simulink model "specifications"  (R2019b)
settings: Solver=FixedStepAuto  StartTime=0.0  StopTime=10.0  FixedStep=fixedStepSize  RelTol=1e-3
settings Model: Creator=JEDDELAN  LastModifiedBy=JEDDELAN
settings DataIOCC: ReturnWorkspaceOutputs=off
settings DebuggingCC: ArithmeticOperatorsInVariantConditions=warning
settings SFSimCC: SimUseLocalCustomCode=off  CustomCodeUndefinedFunction=UseInterfaceOnly
settings RTWCC: RTWUseLocalCustomCode=off

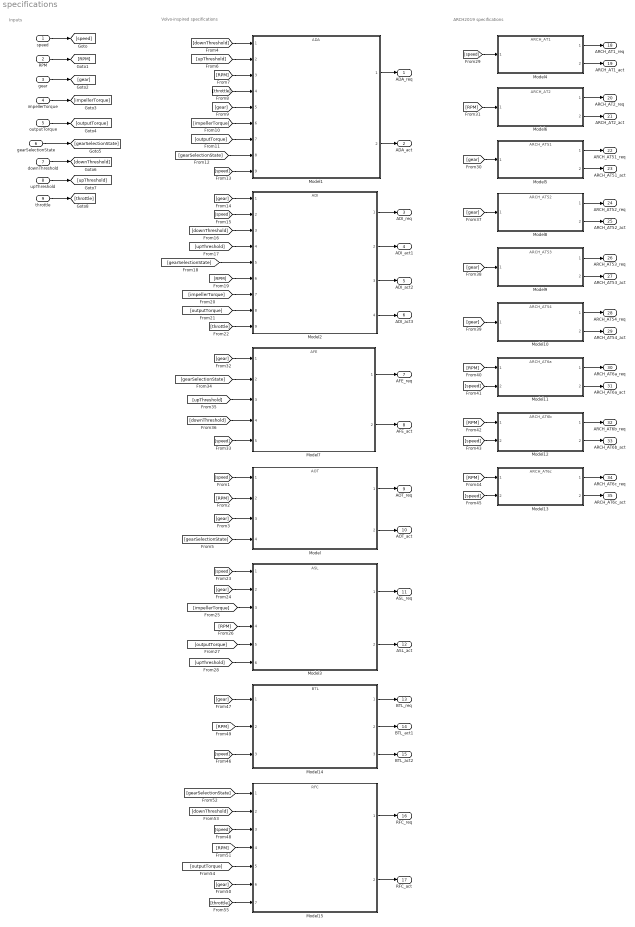
== system specifications ==
  note: Inputs
  note: ARCH2019 specifications
  note: Volvo-inspired specifications
  speed : Inport
  RPM : Inport  Port=2
  gear : Inport  Port=3
  impellerTorque : Inport  Port=4
  outputTorque : Inport  Port=5
  gearSelectionState : Inport  Port=6
  downThreshold : Inport  Port=7  OutDataTypeStr=double
  upThreshold : Inport  Port=8  OutDataTypeStr=double
  throttle : Inport  Port=9
  Model : ModelReference  ModelNameDialog=AOT.slx  SimulationMode=Normal  ModelReferenceVersion=1.170
  Model1 : ModelReference  ModelNameDialog=ADA.slx  SimulationMode=Normal  ModelReferenceVersion=1.259
  Model10 : ModelReference  ModelNameDialog=ARCH_AT54.slx  SimulationMode=Normal  ModelReferenceVersion=1.192
  Model11 : ModelReference  ModelNameDialog=ARCH_AT6a.slx  SimulationMode=Normal  ModelReferenceVersion=1.218
  Model12 : ModelReference  ModelNameDialog=ARCH_AT6b.slx  SimulationMode=Normal  ModelReferenceVersion=1.223
  Model13 : ModelReference  ModelNameDialog=ARCH_AT6c.slx  SimulationMode=Normal  ModelReferenceVersion=1.221
  Model14 : ModelReference  ModelNameDialog=BTL.slx  SimulationMode=Normal  ModelReferenceVersion=1.2366
  Model15 : ModelReference  ModelNameDialog=RFC.slx  SimulationMode=Normal  ModelReferenceVersion=1.2376
  Model2 : ModelReference  ModelNameDialog=ADI.slx  SimulationMode=Normal  ModelReferenceVersion=1.105
  Model3 : ModelReference  ModelNameDialog=ASL.slx  SimulationMode=Normal  ModelReferenceVersion=1.167
  Model4 : ModelReference  ModelNameDialog=ARCH_AT1.slx  SimulationMode=Normal  ModelReferenceVersion=1.161
  Model5 : ModelReference  ModelNameDialog=ARCH_AT51.slx  SimulationMode=Normal  ModelReferenceVersion=1.191
  Model6 : ModelReference  ModelNameDialog=ARCH_AT2.slx  SimulationMode=Normal  ModelReferenceVersion=1.163
  Model7 : ModelReference  ModelNameDialog=AFE.slx  SimulationMode=Normal  ModelReferenceVersion=1.177
  Model8 : ModelReference  ModelNameDialog=ARCH_AT52.slx  SimulationMode=Normal  ModelReferenceVersion=1.193
  Model9 : ModelReference  ModelNameDialog=ARCH_AT53.slx  SimulationMode=Normal  ModelReferenceVersion=1.194
  ADA_req : Outport  VectorParamsAs1DForOutWhenUnconnected=off
  ADA_act : Outport  Port=2  VectorParamsAs1DForOutWhenUnconnected=off
  ADI_req : Outport  Port=3  VectorParamsAs1DForOutWhenUnconnected=off
  ADI_act1 : Outport  Port=4  VectorParamsAs1DForOutWhenUnconnected=off
  ADI_act2 : Outport  Port=5  VectorParamsAs1DForOutWhenUnconnected=off
  ADI_act3 : Outport  Port=6  VectorParamsAs1DForOutWhenUnconnected=off
  AFE_req : Outport  Port=7  VectorParamsAs1DForOutWhenUnconnected=off
  AFE_act : Outport  Port=8  VectorParamsAs1DForOutWhenUnconnected=off
  AOT_req : Outport  Port=9  VectorParamsAs1DForOutWhenUnconnected=off
  AOT_act : Outport  Port=10  VectorParamsAs1DForOutWhenUnconnected=off
  ASL_req : Outport  Port=11  VectorParamsAs1DForOutWhenUnconnected=off
  ASL_act : Outport  Port=12  VectorParamsAs1DForOutWhenUnconnected=off
  BTL_req : Outport  Port=13  VectorParamsAs1DForOutWhenUnconnected=off
  BTL_act1 : Outport  Port=14  VectorParamsAs1DForOutWhenUnconnected=off
  BTL_act2 : Outport  Port=15  VectorParamsAs1DForOutWhenUnconnected=off
  RFC_req : Outport  Port=16  VectorParamsAs1DForOutWhenUnconnected=off
  RFC_act : Outport  Port=17  VectorParamsAs1DForOutWhenUnconnected=off
  ARCH_AT1_req : Outport  Port=18  VectorParamsAs1DForOutWhenUnconnected=off
  ARCH_AT1_act : Outport  Port=19  VectorParamsAs1DForOutWhenUnconnected=off
  ARCH_AT2_req : Outport  Port=20  VectorParamsAs1DForOutWhenUnconnected=off
  ARCH_AT2_act : Outport  Port=21  VectorParamsAs1DForOutWhenUnconnected=off
  ARCH_AT51_req : Outport  Port=22  VectorParamsAs1DForOutWhenUnconnected=off
  ARCH_AT51_act : Outport  Port=23  VectorParamsAs1DForOutWhenUnconnected=off
  ARCH_AT52_req : Outport  Port=24  VectorParamsAs1DForOutWhenUnconnected=off
  ARCH_AT52_act : Outport  Port=25  VectorParamsAs1DForOutWhenUnconnected=off
  ARCH_AT53_req : Outport  Port=26  VectorParamsAs1DForOutWhenUnconnected=off
  ARCH_AT53_act : Outport  Port=27  VectorParamsAs1DForOutWhenUnconnected=off
  ARCH_AT54_req : Outport  Port=28  VectorParamsAs1DForOutWhenUnconnected=off
  ARCH_AT54_act : Outport  Port=29  VectorParamsAs1DForOutWhenUnconnected=off
  ARCH_AT6a_req : Outport  Port=30  VectorParamsAs1DForOutWhenUnconnected=off
  ARCH_AT6a_act : Outport  Port=31  VectorParamsAs1DForOutWhenUnconnected=off
  ARCH_AT6b_req : Outport  Port=32  VectorParamsAs1DForOutWhenUnconnected=off
  ARCH_AT6b_act : Outport  Port=33  VectorParamsAs1DForOutWhenUnconnected=off
  ARCH_AT6c_req : Outport  Port=34  VectorParamsAs1DForOutWhenUnconnected=off
  ARCH_AT6c_act : Outport  Port=35  VectorParamsAs1DForOutWhenUnconnected=off
  wires:
  speed/1 -> [speed]
  [speed] -> Model/1
  RPM/1 -> [RPM]
  gear/1 -> [gear]
  impellerTorque/1 -> [impellerTorque]
  outputTorque/1 -> [outputTorque]
  gearSelectionState/1 -> [gearSelectionState]
  [gear] -> Model/3
  [RPM] -> Model/2
  [gearSelectionState] -> Model/4
  Model/1 -> AOT_req/1
  downThreshold/1 -> [downThreshold]
  upThreshold/1 -> [upThreshold]
  Model/2 -> AOT_act/1
  [gear] -> Model1/5
  [impellerTorque] -> Model1/6
  [outputTorque] -> Model1/7
  [gearSelectionState] -> Model1/8
  [speed] -> Model1/9
  [throttle] -> Model1/4
  [RPM] -> Model1/3
  [upThreshold] -> Model1/2
  [downThreshold] -> Model1/1
  throttle/1 -> [throttle]
  Model1/1 -> ADA_req/1
  Model1/2 -> ADA_act/1
  [gear] -> Model2/1
  [speed] -> Model2/2
  [downThreshold] -> Model2/3
  [throttle] -> Model2/9
  [outputTorque] -> Model2/8
  [impellerTorque] -> Model2/7
  [RPM] -> Model2/6
  [gearSelectionState] -> Model2/5
  [upThreshold] -> Model2/4
  Model2/1 -> ADI_req/1
  Model2/4 -> ADI_act3/1
  Model2/3 -> ADI_act2/1
  Model2/2 -> ADI_act1/1
  [speed] -> Model3/1
  [gear] -> Model3/2
  [impellerTorque] -> Model3/3
  [RPM] -> Model3/4
  [outputTorque] -> Model3/5
  [upThreshold] -> Model3/6
  Model3/1 -> ASL_req/1
  Model3/2 -> ASL_act/1
  [speed] -> Model4/1
  Model4/1 -> ARCH_AT1_req/1
  Model4/2 -> ARCH_AT1_act/1
  [gear] -> Model5/1
  Model5/1 -> ARCH_AT51_req/1
  Model6/1 -> ARCH_AT2_req/1
  [RPM] -> Model6/1
  Model6/2 -> ARCH_AT2_act/1
  [gear] -> Model7/1
  [speed] -> Model7/5
  [upThreshold] -> Model7/3
  [downThreshold] -> Model7/4
  Model7/1 -> AFE_req/1
  Model7/2 -> AFE_act/1
  Model5/2 -> ARCH_AT51_act/1
  Model8/2 -> ARCH_AT52_act/1
  Model8/1 -> ARCH_AT52_req/1
  [gear] -> Model8/1
  Model9/2 -> ARCH_AT53_act/1
  Model9/1 -> ARCH_AT53_req/1
  [gear] -> Model9/1
  Model10/2 -> ARCH_AT54_act/1
  Model10/1 -> ARCH_AT54_req/1
  [gear] -> Model10/1
  [gearSelectionState] -> Model7/2
  Model11/2 -> ARCH_AT6a_act/1
  Model11/1 -> ARCH_AT6a_req/1
  [RPM] -> Model11/1
  [speed] -> Model11/2
  Model12/1 -> ARCH_AT6b_req/1
  Model12/2 -> ARCH_AT6b_act/1
  [speed] -> Model12/2
  [RPM] -> Model12/1
  Model13/1 -> ARCH_AT6c_req/1
  Model13/2 -> ARCH_AT6c_act/1
  [speed] -> Model13/2
  [RPM] -> Model13/1
  [RPM] -> Model14/2
  [gear] -> Model14/1
  Model14/2 -> BTL_act1/1
  Model14/1 -> BTL_req/1
  [speed] -> Model14/3
  Model14/3 -> BTL_act2/1
  Model15/2 -> RFC_act/1
  Model15/1 -> RFC_req/1
  [gearSelectionState] -> Model15/1
  [downThreshold] -> Model15/2
  [speed] -> Model15/3
  [gear] -> Model15/6
  [RPM] -> Model15/4
  [outputTorque] -> Model15/5
  [throttle] -> Model15/7
